simulink library "INT_AirSys_AirTemp"  (R2016b)
settings: Solver=VariableStepAuto  StartTime=0.0  StopTime=10.0  RelTol=1e-3
settings Model: Creator=Administrator  LastModifiedBy=Administrator

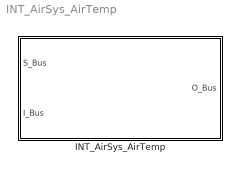
== system INT_AirSys_AirTemp ==
  INT_AirSys_AirTemp : Subsystem

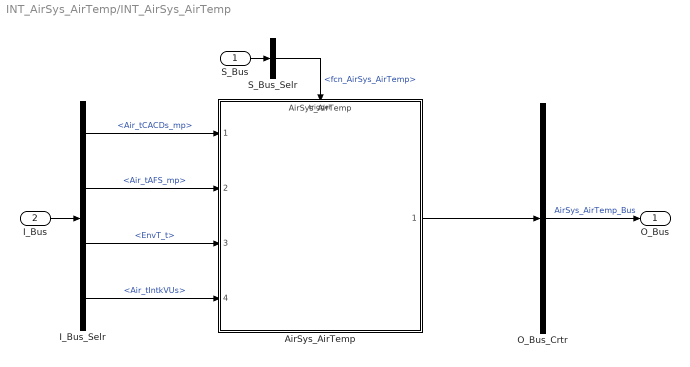
== system INT_AirSys_AirTemp/INT_AirSys_AirTemp ==
  S_Bus : Inport
  I_Bus : Inport  Port=2
  AirSys_AirTemp : ModelReference  ModelNameDialog=AirSys_AirTemp  SimulationMode=Normal  ModelReferenceVersion=1.3  TriggerPortName=function  TriggerPortTriggerType=function-call  TriggerPortStatesWhenEnabling=held
  I_Bus_Selr : BusSelector  OutputSignals=Air_tCACDs_mp,Air_tAFS_mp,EnvT_t,Air_tIntkVUs
  O_Bus_Crtr : BusCreator  Inputs=1
  S_Bus_Selr : BusSelector  OutputSignals=fcn_AirSys_AirTemp
  O_Bus : Outport
  wires:
  S_Bus_Selr/1 -> AirSys_AirTemp/Trigger  "<fcn_AirSys_AirTemp>"
  S_Bus/1 -> S_Bus_Selr/1
  I_Bus/1 -> I_Bus_Selr/1
  I_Bus_Selr/1 -> AirSys_AirTemp/1  "<Air_tCACDs_mp>"
  I_Bus_Selr/2 -> AirSys_AirTemp/2  "<Air_tAFS_mp>"
  I_Bus_Selr/3 -> AirSys_AirTemp/3  "<EnvT_t>"
  I_Bus_Selr/4 -> AirSys_AirTemp/4  "<Air_tIntkVUs>"
  O_Bus_Crtr/1 -> O_Bus/1  "AirSys_AirTemp_Bus"
  AirSys_AirTemp/1 -> O_Bus_Crtr/1
